simulink model "Immersion_Invariance"  (R2020b)
settings: Solver=FixedStepAuto  StartTime=0.0  StopTime=10.0  FixedStep=DT  RelTol=1e-3
undefined symbols (not defined in the file or in its folder): C_d, CP, CP_lambda, CP_theta, II_gamma, II_phi0, II_vx0, J_r, K_d, PR_A, PR_B, PR_C, PR_L, PR_theta0, R, rho
settings Model: Creator=lpwoolcock  LastModifiedBy=lpwoolcock

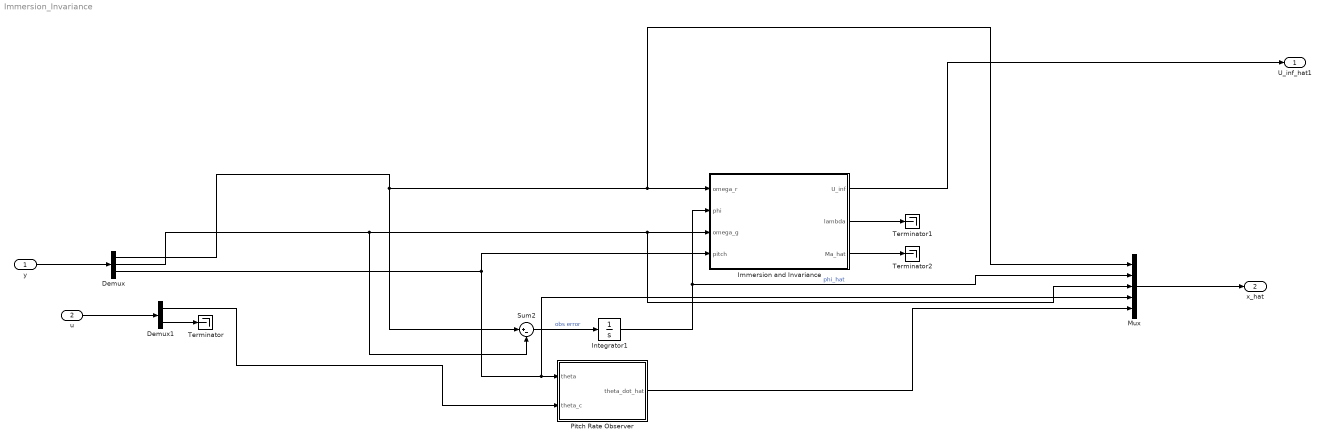
== system Immersion_Invariance ==
  y : Inport  PortDimensions=[3 1]
  u : Inport  Port=2  PortDimensions=[2 1]
  Demux : Demux  Outputs=3
  Demux1 : Demux  Outputs=2
  Immersion and Invariance : Subsystem  TreatAsAtomicUnit=on
  Integrator1 : Integrator  InitialCondition=II_phi0
  Mux : Mux  Inputs=5
  Pitch Rate Observer : Subsystem  TreatAsAtomicUnit=on
  Sum2 : Sum  Inputs=|+-
  Terminator : Terminator
  Terminator1 : Terminator
  Terminator2 : Terminator
  U_inf_hat1 : Outport  PortDimensions=1
  x_hat : Outport  Port=2  PortDimensions=[5 1]
  wires:
  Sum2/1 -> Integrator1/1  "obs error"
  Demux/3 -> Immersion and Invariance/4(pitch), Mux/4, Pitch Rate Observer/1(theta)
  Integrator1/1 -> Mux/2, Immersion and Invariance/2(phi)  "phi_hat"
  Demux/1 -> Mux/1, Immersion and Invariance/1(omega_r), Sum2/1
  Demux/2 -> Mux/3, Immersion and Invariance/3(omega_g), Sum2/2
  Demux1/1 -> Pitch Rate Observer/2(theta_c)
  y/1 -> Demux/1
  u/1 -> Demux1/1
  Mux/1 -> x_hat/1
  Immersion and Invariance/1(U_inf) -> U_inf_hat1/1
  Pitch Rate Observer/1(theta_dot_hat) -> Mux/5
  Demux1/2 -> Terminator/1
  Immersion and Invariance/2(lambda) -> Terminator1/1
  Immersion and Invariance/3(Ma_hat) -> Terminator2/1

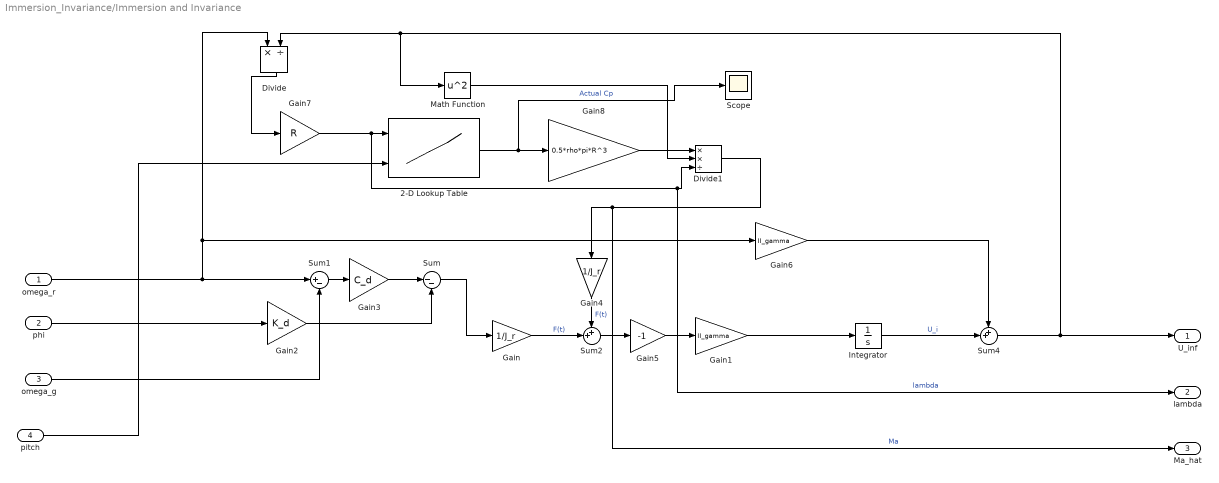
== system Immersion_Invariance/Immersion and Invariance ==
  omega_r : Inport
  phi : Inport  Port=2
  omega_g : Inport  Port=3
  pitch : Inport  Port=4
  2-D Lookup Table : Lookup_n-D  BreakpointsForDimension1=CP_lambda  BreakpointsForDimension2=CP_theta  Table=CP  InterpMethod=Cubic spline  ExtrapMethod=Cubic spline  InternalRulePriority=Speed  RndMeth=Simplest  InputSameDT=on
      settings: InputPortMap=u0,u1
  Divide : Product  Inputs=*/
  Divide1 : Product  Inputs=**/
  Gain : Gain  Gain=1/J_r
  Gain1 : Gain  Gain=II_gamma
  Gain2 : Gain  Gain=K_d
  Gain3 : Gain  Gain=C_d
  Gain4 : Gain  Gain=1/J_r
  Gain5 : Gain  Gain=-1
  Gain6 : Gain  Gain=II_gamma
  Gain7 : Gain  Gain=R
  Gain8 : Gain  Gain=0.5*rho*pi*R^3
  Integrator : Integrator  InitialCondition=II_vx0
  Math Function : Math  Operator=square  SaturateOnIntegerOverflow=on
  Scope : Scope
  Sum : Sum  Inputs=|--
  Sum1 : Sum  Inputs=|+-
  Sum2 : Sum  Inputs=++|
  Sum4 : Sum  Inputs=++|
  U_inf : Outport
  lambda : Outport  Port=2
  Ma_hat : Outport  Port=3
  wires:
  phi/1 -> Gain2/1
  Gain2/1 -> Sum/2
  omega_g/1 -> Sum1/2
  Sum1/1 -> Gain3/1
  Gain3/1 -> Sum/1
  Sum/1 -> Gain/1
  omega_r/1 -> Sum1/1, Divide/1, Gain6/1
  Gain/1 -> Sum2/2  "F(t)"
  Gain4/1 -> Sum2/1  "F(t)"
  Sum2/1 -> Gain5/1
  Gain5/1 -> Gain1/1
  Integrator/1 -> Sum4/2  "U_i"
  Gain1/1 -> Integrator/1
  Gain6/1 -> Sum4/1
  pitch/1 -> 2-D Lookup Table/2
  Gain7/1 -> lambda/1, Divide1/3, 2-D Lookup Table/1  "lambda"
  Divide/1 -> Gain7/1
  Gain8/1 -> Divide1/1
  Divide1/1 -> Ma_hat/1, Gain4/1  "Ma"
  Math Function/1 -> Divide1/2
  2-D Lookup Table/1 -> Scope/1, Gain8/1  "Actual Cp"
  Sum4/1 -> Math Function/1, Divide/2, U_inf/1

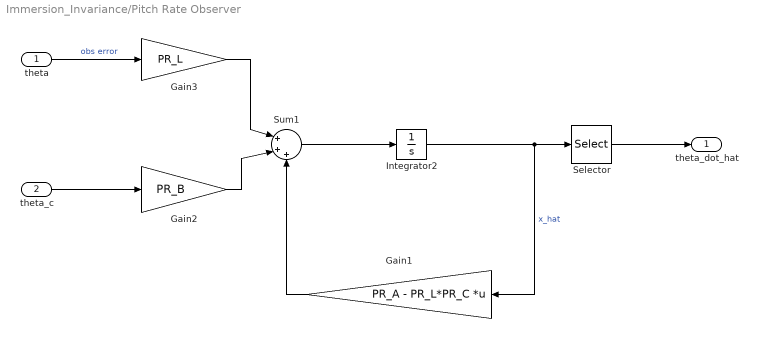
== system Immersion_Invariance/Pitch Rate Observer ==
  theta : Inport
  theta_c : Inport  Port=2
  Gain1 : Gain  Gain=PR_A - PR_L*PR_C  Multiplication=Matrix(K*u)
  Gain2 : Gain  Gain=PR_B
  Gain3 : Gain  Gain=PR_L
  Integrator2 : Integrator  InitialCondition=PR_theta0
  Selector : Selector  InputPortWidth=2  IndexOptions=Index vector (dialog)  Indices=[2]  OutputSizes=1
  Sum1 : Sum  Inputs=|+++
  theta_dot_hat : Outport
  wires:
  Sum1/1 -> Integrator2/1
  Gain2/1 -> Sum1/2
  Gain3/1 -> Sum1/1
  Integrator2/1 -> Selector/1, Gain1/1  "x_hat"
  theta/1 -> Gain3/1  "obs error"
  Gain1/1 -> Sum1/3
  theta_c/1 -> Gain2/1
  Selector/1 -> theta_dot_hat/1
